simulink model "model4"  (R2024b)
settings: Solver=VariableStepAuto  StartTime=0.0  StopTime=10.0  RelTol=1e-3
undefined symbols (not defined in the file): A1, A2, c1, c2
settings Model: Creator=kacpe  LastModifiedBy=kacpe

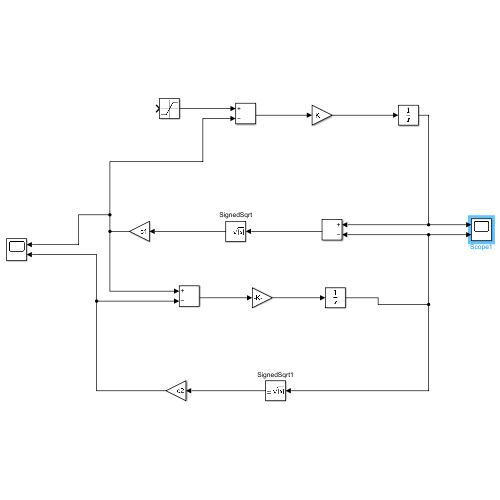
[thumbnail: Simulink's stored preview of the top-level diagram]
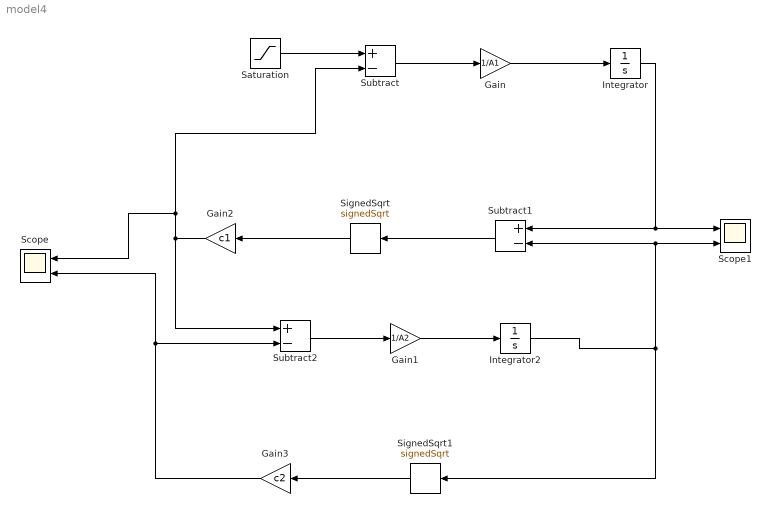
== system model4 ==
  Gain : Gain  Gain=1/A1
  Gain1 : Gain  Gain=1/A2
  Gain2 : Gain  Gain=c1
  Gain3 : Gain  Gain=c2
  Integrator : Integrator
  Integrator2 : Integrator
  Saturation : Saturate
  Scope : Scope  NumInputPorts=2
  Scope1 : Scope  NumInputPorts=2
  SignedSqrt : Sqrt  Operator=signedSqrt  IntermediateResultsDataTypeStr=single
  SignedSqrt1 : Sqrt  Operator=signedSqrt  IntermediateResultsDataTypeStr=single
  Subtract : Sum  Inputs=+-
  Subtract1 : Sum  Inputs=+-
  Subtract2 : Sum  Inputs=+-
  wires:
  Saturation/1 -> Subtract/1
  Subtract/1 -> Gain/1
  Gain/1 -> Integrator/1
  Integrator/1 -> Subtract1/1, Scope1/1
  Integrator2/1 -> Scope1/2, Subtract1/2, SignedSqrt1/1
  Gain3/1 -> Subtract2/2, Scope/2
  Gain2/1 -> Subtract2/1, Subtract/2, Scope/1
  Subtract2/1 -> Gain1/1
  Gain1/1 -> Integrator2/1
  SignedSqrt/1 -> Gain2/1
  Subtract1/1 -> SignedSqrt/1
  SignedSqrt1/1 -> Gain3/1
